simulink model "quadrotor_altitude_tracking"  (R2024b)
settings: Solver=VariableStepAuto  StartTime=0.0  StopTime=simulation_time  RelTol=1e-3
values from neighbouring files (symbols this model uses):
  initial_height = 0    [quadrotor_altitude_tracking_settings.m]
  initial_velocity = 0    [quadrotor_altitude_tracking_settings.m]
  Kd = 2    [quadrotor_altitude_tracking_settings.m]
  Kp = 5    [quadrotor_altitude_tracking_settings.m]
libraries: uavutilslib x1
settings Model: Creator=zhes  LastModifiedBy=zhes
settings ConfigSetCC: ModbusTableInfo=[]

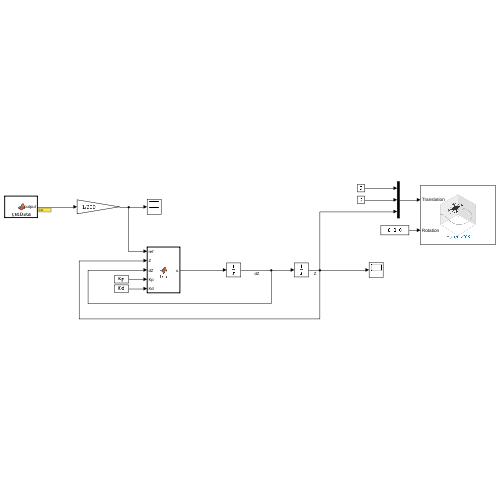
[thumbnail: Simulink's stored preview of the top-level diagram]
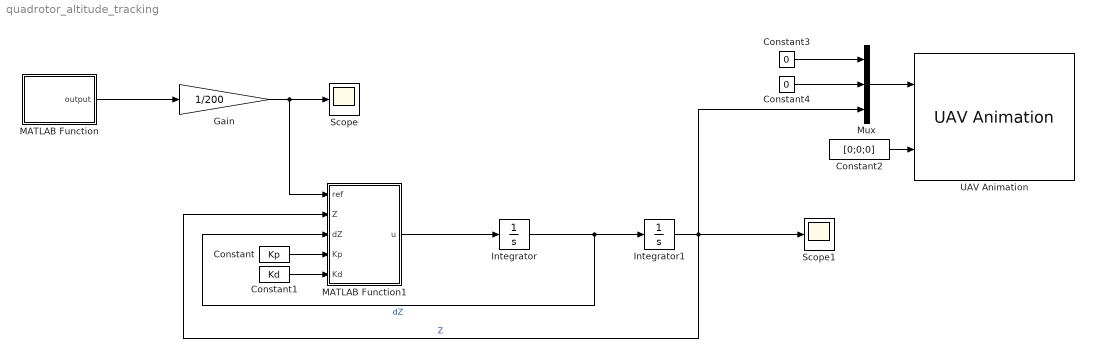
== system quadrotor_altitude_tracking ==
  Constant : Constant  Value=Kp
  Constant1 : Constant  Value=Kd
  Constant2 : Constant  Value=[0;0;0]
  Constant3 : Constant  Value=0
  Constant4 : Constant  Value=0
  Gain : Gain  Gain=1/200
  Integrator : Integrator  InitialCondition=initial_velocity
  Integrator1 : Integrator  InitialCondition=initial_height
  MATLAB Function : MATLAB Function  TreatAsAtomicUnit=on
  MATLAB Function1 : MATLAB Function  TreatAsAtomicUnit=on
  Mux : Mux  Inputs=3
  Scope : Scope
  Scope1 : Scope
  UAV Animation : uavutilslib/UAV Animation  NumUAV=1  DynamicUAVConfig=off  UAVType=Multirotor  UAVSize=1  UAVColor=[1 0 0]  UAVTrajectoryAlpha=1  InertialZDirection=Up  RotationFormat=Euler ZYX  DrawMarkers=off  SampleTime=-1
  wires:
  MATLAB Function/1(output) -> Gain/1
  Gain/1 -> MATLAB Function1/1(ref), Scope/1
  Integrator/1 -> MATLAB Function1/3(dZ), Integrator1/1  "dZ"
  MATLAB Function1/1(u) -> Integrator/1
  Integrator1/1 -> Mux/3, Scope1/1, MATLAB Function1/2(Z)  "Z"
  Constant/1 -> MATLAB Function1/4(Kp)
  Constant1/1 -> MATLAB Function1/5(Kd)
  Constant2/1 -> UAV Animation/2
  Mux/1 -> UAV Animation/1
  Constant4/1 -> Mux/2
  Constant3/1 -> Mux/1

== matlab function quadrotor_altitude_tracking/MATLAB Function1 ==
  data: ref input; u output; Z input; dZ input; Kp input; Kd input
function u = fcn(ref, Z, dZ, Kp, Kd)

u = Kp * (ref - Z) + Kd * (0 - dZ);

== matlab function quadrotor_altitude_tracking/MATLAB Function ==
  data: output output
function output = getData()
    output = 0;
    coder.extrinsic('evalin');
    data = evalin('base', 'reference');
    output = data; % 输出最新值
end
